simulink subsystem "PID_Controller_Subsystem"  (R2023a)
settings: Solver=VariableStepAuto  StartTime=0.0  StopTime=10.0  RelTol=1e-3

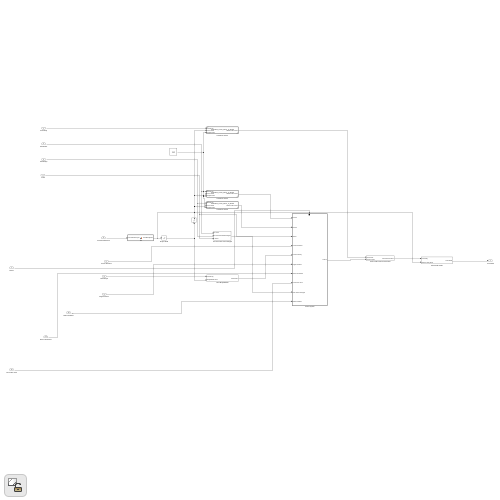
[thumbnail: Simulink's stored preview of the top-level diagram]
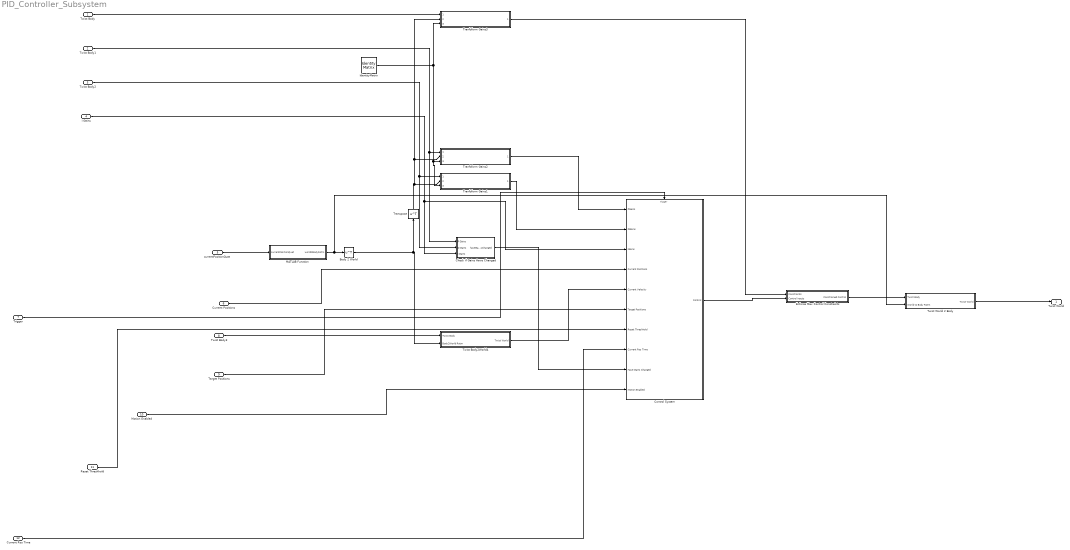
== system PID_Controller_Subsystem ==
  Twist Body : Inport
  Twist Body1 : Inport  Port=2
  Twist Body2 : Inport  Port=3
  I Gains : Inport  Port=4
  currentPositionQuat : Inport  Port=5
  Current Positions : Inport  Port=6
  Trigger : Inport  Port=7
  Twist Body3 : Inport  Port=8
  Target Positions : Inport  Port=9
  Motion Enabled : Inport  Port=10
  Reset Threshhold : Inport  Port=11
  Current Ros Time : Inport  Port=12
  Body 2 World : Math  Operator=transpose
  Check if Gains Have Changed : Subsystem
  Control System : Subsystem
  Enforce Max Control Constraints : Subsystem
  IdentityMatrix : IdentityMatrix  OutputDimensions=3
  MATLAB Function : MATLAB Function  TreatAsAtomicUnit=on
  Tranfsform Gains1 : Subsystem  TreatAsAtomicUnit=on  ReferencedSubsystem=Tranfsform_Linear_Gains_To_World
  Tranfsform Gains2 : Subsystem  TreatAsAtomicUnit=on  ReferencedSubsystem=Tranfsform_Linear_Gains_To_World
  Tranfsform Gains3 : Subsystem  TreatAsAtomicUnit=on  ReferencedSubsystem=Tranfsform_Linear_Gains_To_World
  Transpose : Math  Operator=transpose
  Twist Body2World4 : Subsystem
  Twist World 2 Body : Subsystem
  Twist World : Outport
  wires:
  Tranfsform Gains2/1 -> Control System/1(PGains)
  Target Positions/1 -> Control System/6(Target Positions)
  Control System/1(Control) -> Enforce Max Control Constraints/2(Control Inputs)
  MATLAB Function/1(world2BodyRotm) -> Body 2 World/1, Twist World 2 Body/2(World to Body Rotm)
  Tranfsform Gains3/1 -> Enforce Max Control Constraints/1(Constraints)
  Twist Body1/1 -> Check if Gains Have Changed/1(P Gains), Tranfsform Gains2/1
  Tranfsform Gains1/1 -> Control System/2(DGains)
  IdentityMatrix/1 -> Tranfsform Gains2/3, Tranfsform Gains1/3, Tranfsform Gains3/3
  Enforce Max Control Constraints/1(Constrained Control) -> Twist World 2 Body/1(Twist Body)
  Check if Gains Have Changed/1(haveGainsChanged) -> Control System/9(Have Gains Changed)
  Reset Threshhold/1 -> Control System/7(Reset Threshhold)
  Current Positions/1 -> Control System/4(Current Positions)
  Current Ros Time/1 -> Control System/8(Current Ros Time)
  Twist Body3/1 -> Twist Body2World4/1(Twist Body)
  Twist Body2World4/1(Twist World) -> Control System/5(Current Velocity)
  currentPositionQuat/1 -> MATLAB Function/1(currentPositionQuat)
  Twist World 2 Body/1(Twist World) -> Twist World/1
  Twist Body2/1 -> Check if Gains Have Changed/2(D Gains), Tranfsform Gains1/1
  Twist Body/1 -> Tranfsform Gains3/1
  Motion Enabled/1 -> Control System/10(Motion Enabled)
  I Gains/1 -> Control System/3(IGains), Check if Gains Have Changed/3(I Gains)
  Body 2 World/1 -> Transpose/1, Twist Body2World4/2(Body2World Rotm)
  Transpose/1 -> Tranfsform Gains3/2, Tranfsform Gains2/2, Tranfsform Gains1/2
  Trigger/1 -> Control System/Trigger

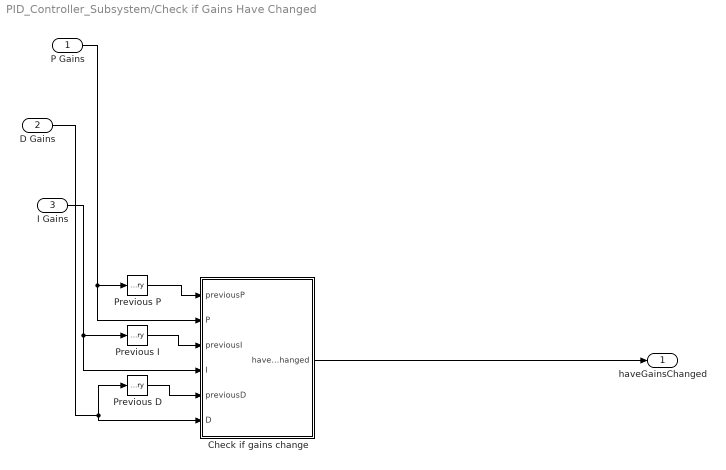
== system PID_Controller_Subsystem/Check if Gains Have Changed ==
  P Gains : Inport
  D Gains : Inport  Port=2
  I Gains : Inport  Port=3
  Check if gains change : MATLAB Function  TreatAsAtomicUnit=on
  Previous D : Memory  InheritSampleTime=on
  Previous I : Memory  InheritSampleTime=on
  Previous P : Memory  InheritSampleTime=on
  haveGainsChanged : Outport
  wires:
  Check if gains change/1(haveGainsChanged) -> haveGainsChanged/1
  D Gains/1 -> Check if gains change/6(D), Previous D/1
  Previous D/1 -> Check if gains change/5(previousD)
  P Gains/1 -> Previous P/1, Check if gains change/2(P)
  Previous P/1 -> Check if gains change/1(previousP)
  Previous I/1 -> Check if gains change/3(previousI)
  I Gains/1 -> Previous I/1, Check if gains change/4(I)

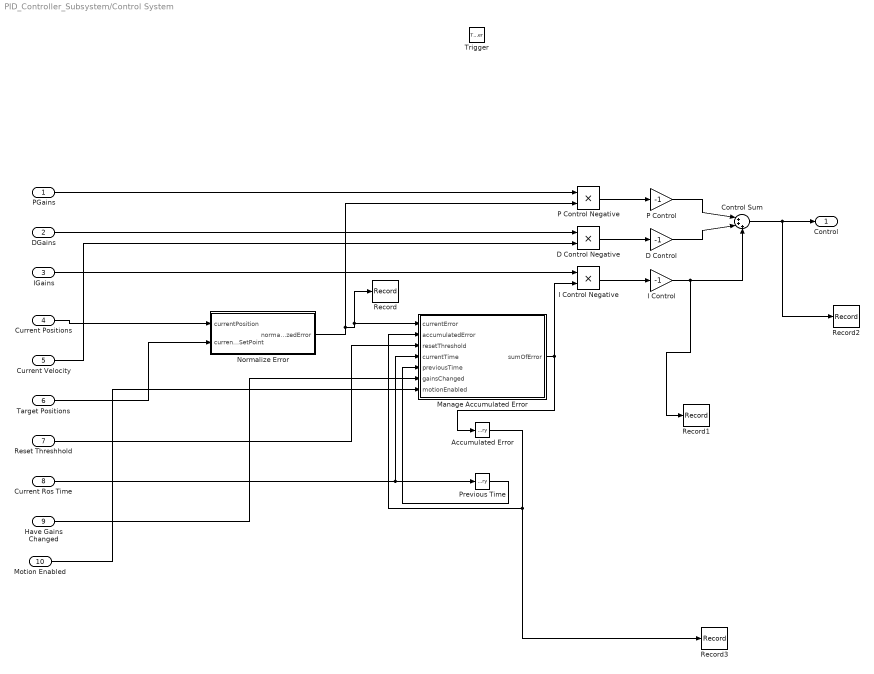
== system PID_Controller_Subsystem/Control System ==
  PGains : Inport
  DGains : Inport  Port=2
  IGains : Inport  Port=3
  Current Positions : Inport  Port=4
  Current Velocity : Inport  Port=5
  Target Positions : Inport  Port=6
  Reset Threshhold : Inport  Port=7
  Current Ros Time : Inport  Port=8
  Have Gains Changed : Inport  Port=9
  Motion Enabled : Inport  Port=10
  Trigger : TriggerPort  VariantControl=(inherit)  PortDimensions=1
  Accumulated Error : Memory  InheritSampleTime=on
  Control Sum : Sum  Inputs=|+++
  D Control : Gain  Gain=-1
  D Control Negative : Product
  I Control : Gain  Gain=-1
  I Control Negative : Product
  Manage Accumulated Error : MATLAB Function  TreatAsAtomicUnit=on
  Normalize Error : MATLAB Function  TreatAsAtomicUnit=on
  P Control : Gain  Gain=-1
  P Control Negative : Product
  Previous Time : Memory  InitialCondition=-1  InheritSampleTime=on
  Record{,1..3} (4 alike) : Record  FileSettingsInternal="{\"entries\":[{\"content\":{\"excelSettings\":{\"content\":{},\"type\":\"Streamout.ExcelSettings\"}},\"type\":\"Streamout.FileSettingStorage\",\"uuid\":\"\"}],\"packageUris\":[\"http:\\/\\/schema.mathworks.com\\/mf0\\/streamout_blocks\\/R2020a\"],\"version\":\"1.0\"}"  Layout=[1 1]  SignalsInternal="{\"entries\":[{\"content\":{},\"type\":\"RecordBlkView.InputSignals\",\"uuid\":\"\"}],\"packageUris\":[\"http:\\/\\/schema.mathworks.com\\/mf0\\/streamout_blocks\\/R2020a\"],\"version\":\"1.0\"}"  VisualizationBindings="{\"sparklinesplugin\":{\"info\":[{\"bindingParametersList\":[],\"subplotID\":1}]}}"
  Control : Outport
  wires:
  Motion Enabled/1 -> Manage Accumulated Error/7(motionEnabled)
  Target Positions/1 -> Normalize Error/2(currentSetPoint)
  Have Gains Changed/1 -> Manage Accumulated Error/6(gainsChanged)
  DGains/1 -> D Control Negative/1
  PGains/1 -> P Control Negative/1
  IGains/1 -> I Control Negative/1
  Current Ros Time/1 -> Manage Accumulated Error/4(currentTime), Previous Time/1
  Previous Time/1 -> Manage Accumulated Error/5(previousTime)
  Normalize Error/1(normalizedError) -> Manage Accumulated Error/1(currentError), Record/1, P Control Negative/2
  Current Positions/1 -> Normalize Error/1(currentPosition)
  Control Sum/1 -> Control/1, Record2/1
  I Control Negative/1 -> I Control/1
  Manage Accumulated Error/1(sumOfError) -> I Control Negative/2, Accumulated Error/1
  D Control/1 -> Control Sum/2
  Accumulated Error/1 -> Manage Accumulated Error/2(accumulatedError), Record3/1
  P Control Negative/1 -> P Control/1
  D Control Negative/1 -> D Control/1
  P Control/1 -> Control Sum/1
  Current Velocity/1 -> D Control Negative/2
  I Control/1 -> Control Sum/3, Record1/1
  Reset Threshhold/1 -> Manage Accumulated Error/3(resetThreshold)

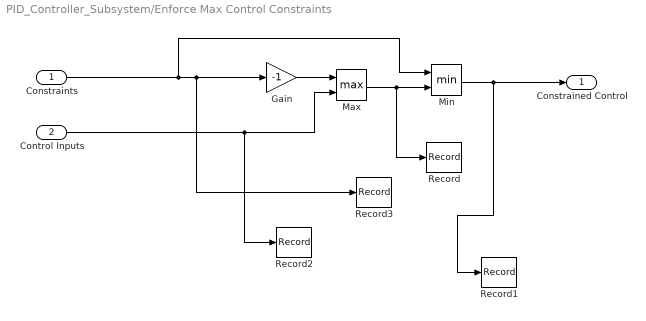
== system PID_Controller_Subsystem/Enforce Max Control Constraints ==
  Constraints : Inport
  Control Inputs : Inport  Port=2
  Gain : Gain  Gain=-1
  Max : MinMax  Function=max  Inputs=2
  Min : MinMax  Inputs=2
  Record{,1..3} (4 alike) : Record  FileSettingsInternal="{\"entries\":[{\"content\":{\"excelSettings\":{\"content\":{},\"type\":\"Streamout.ExcelSettings\"}},\"type\":\"Streamout.FileSettingStorage\",\"uuid\":\"\"}],\"packageUris\":[\"http:\\/\\/schema.mathworks.com\\/mf0\\/streamout_blocks\\/R2020a\"],\"version\":\"1.0\"}"  Layout=[1 1]  SignalsInternal="{\"entries\":[{\"content\":{},\"type\":\"RecordBlkView.InputSignals\",\"uuid\":\"\"}],\"packageUris\":[\"http:\\/\\/schema.mathworks.com\\/mf0\\/streamout_blocks\\/R2020a\"],\"version\":\"1.0\"}"  VisualizationBindings="{\"sparklinesplugin\":{\"info\":[{\"bindingParametersList\":[],\"subplotID\":1}]}}"
  Constrained Control : Outport
  wires:
  Constraints/1 -> Gain/1, Record3/1, Min/1
  Max/1 -> Min/2, Record/1
  Control Inputs/1 -> Max/2, Record2/1
  Min/1 -> Constrained Control/1, Record1/1
  Gain/1 -> Max/1

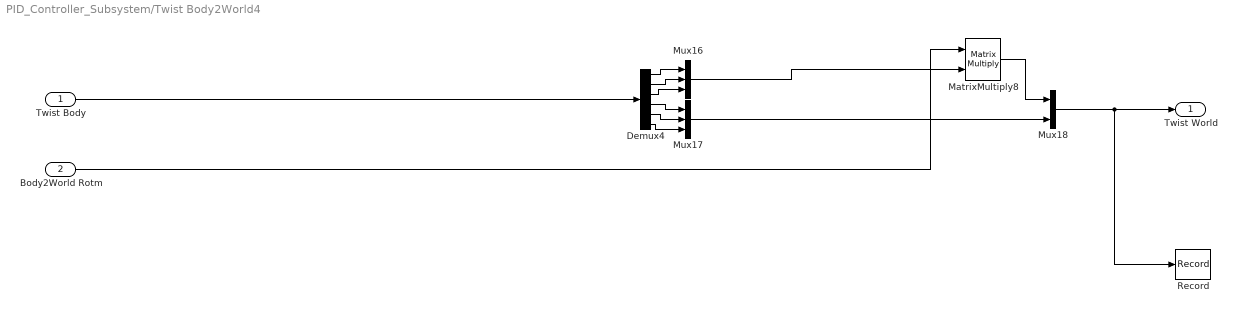
== system PID_Controller_Subsystem/Twist Body2World4 ==
  Twist Body : Inport
  Body2World Rotm : Inport  Port=2
  Demux4 : Demux  Outputs=6
  MatrixMultiply8 : Product  Multiplication=Matrix(*)
  Mux16 : Mux  Inputs=3
  Mux17 : Mux  Inputs=3
  Mux18 : Mux  Inputs=2
  Record : Record  FileSettingsInternal="{\"entries\":[{\"content\":{\"excelSettings\":{\"content\":{},\"type\":\"Streamout.ExcelSettings\"}},\"type\":\"Streamout.FileSettingStorage\",\"uuid\":\"\"}],\"packageUris\":[\"http:\\/\\/schema.mathworks.com\\/mf0\\/streamout_blocks\\/R2020a\"],\"version\":\"1.0\"}"  Layout=[1 1]  SignalsInternal="{\"entries\":[{\"content\":{},\"type\":\"RecordBlkView.InputSignals\",\"uuid\":\"\"}],\"packageUris\":[\"http:\\/\\/schema.mathworks.com\\/mf0\\/streamout_blocks\\/R2020a\"],\"version\":\"1.0\"}"  VisualizationBindings="{\"sparklinesplugin\":{\"info\":[{\"bindingParametersList\":[],\"subplotID\":1}]}}"
  Twist World : Outport
  wires:
  Mux18/1 -> Twist World/1, Record/1
  MatrixMultiply8/1 -> Mux18/1
  Body2World Rotm/1 -> MatrixMultiply8/1
  Demux4/3 -> Mux16/3
  Twist Body/1 -> Demux4/1
  Mux17/1 -> Mux18/2
  Demux4/5 -> Mux17/2
  Demux4/1 -> Mux16/1
  Demux4/6 -> Mux17/3
  Mux16/1 -> MatrixMultiply8/2
  Demux4/4 -> Mux17/1
  Demux4/2 -> Mux16/2

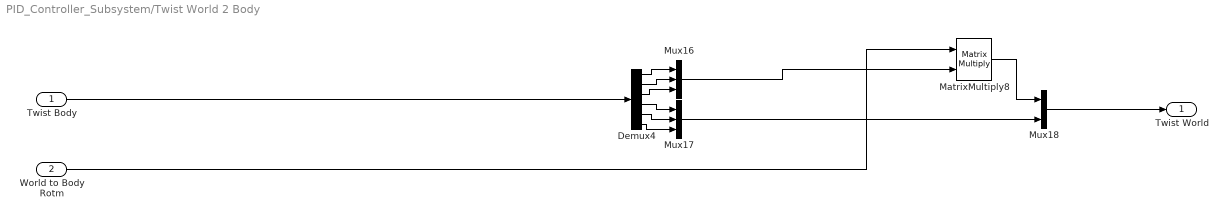
== system PID_Controller_Subsystem/Twist World 2 Body ==
  Twist Body : Inport
  World to Body Rotm : Inport  Port=2
  Demux4 : Demux  Outputs=6
  MatrixMultiply8 : Product  Multiplication=Matrix(*)
  Mux16 : Mux  Inputs=3
  Mux17 : Mux  Inputs=3
  Mux18 : Mux  Inputs=2
  Twist World : Outport
  wires:
  World to Body Rotm/1 -> MatrixMultiply8/1
  Mux18/1 -> Twist World/1
  MatrixMultiply8/1 -> Mux18/1
  Demux4/3 -> Mux16/3
  Twist Body/1 -> Demux4/1
  Mux17/1 -> Mux18/2
  Demux4/5 -> Mux17/2
  Demux4/1 -> Mux16/1
  Demux4/6 -> Mux17/3
  Mux16/1 -> MatrixMultiply8/2
  Demux4/4 -> Mux17/1
  Demux4/2 -> Mux16/2

== matlab function PID_Controller_Subsystem/Control System/Manage Accumulated Error ==
function sumOfError = fcn(currentError, accumulatedError, resetThreshold, currentTime, previousTime, gainsChanged, motionEnabled)

deltaTime = 0;
if(previousTime <= 0)
    sumOfError = zeros(1,6);
    return 
else
    deltaTime = currentTime - previousTime;
end

sum = zeros(1,6);

%if gains get reset, reset accumulator
if(gainsChanged || ~motionEnabled)
   sumOfError = zeros(1,6);

   disp(gainsChanged)

   return
end

%check each degree of freedom
for i = 1:6
    sum(i) = (currentError(i)) * deltaTime + accumulatedError(i);

    if(currentError(i) > resetThreshold)
        sum(i) = 0;
    end

    %reset if nan
    if(isnan(currentError(i)))
        sum(i) = 0;
    end

end

sumOfError = sum;

== matlab function PID_Controller_Subsystem/Control System/Normalize Error ==
function normalizedError = fcn(currentPosition, currentSetPoint)

normalized = zeros(1,6);

normalized(1) = currentPosition(1) - currentSetPoint(1);
normalized(2) = currentPosition(2) - currentSetPoint(2);
normalized(3) = currentPosition(3) - currentSetPoint(3);

W2B = [currentPosition(7), currentPosition(4), currentPosition(5), currentPosition(6)];
setQuat = [currentSetPoint(7), -currentSetPoint(4), -currentSetPoint(5), -currentSetPoint(6)];


%Talos Heading in Body Frame
Tbody = [1,0,0,0];

%Transform from Body 2 World
B2W = [W2B(1), -W2B(2), -W2B(3), -W2B(4)] / (norm(W2B) ^ 2);

%Talos Heading in World Frame
TWorld = quatmultiply(Tbody, B2W);

%Talos Heading in World Frame Conjugate
TWorldI = [TWorld(1), -TWorld(2), -TWorld(3), -TWorld(4)];

disp(TWorld)

%Current Yaw Error
eQuat = quatmultiply(setQuat, TWorldI);

% %axis Error
axisError = [eQuat(2), eQuat(3), eQuat(4)];
if(eQuat(1) < 0)
    axisError = -axisError;
end


normalized(4) = axisError(1);
normalized(5) = axisError(2);
normalized(6) = axisError(3);

normalizedError = normalized;

== matlab function PID_Controller_Subsystem/MATLAB Function ==
function world2BodyRotm = fcn(currentPositionQuat)


world2BodyRotm = quat2rotm([currentPositionQuat(7), currentPositionQuat(4), currentPositionQuat(5), currentPositionQuat(6)]);

%fuk u matlab
world2BodyRotm = transpose(world2BodyRotm);

== matlab function PID_Controller_Subsystem/Check if Gains Have Changed/Check if gains change ==
function haveGainsChanged  = fcn(previousP, P, previousI, I, previousD, D)


%check if P gains have changed
if(~isequal(P, previousP))
    haveGainsChanged = true;
    return
end


%check if  I gains have changed
if(~isequal(I, previousI))
    haveGainsChanged = true;
    return
end


%check if  D gains have changed
if(~isequal(D, previousD))
    haveGainsChanged = true;
    return
end

haveGainsChanged = false;
